simulink model "Anticipativo"  (R2018a)
settings: Solver=VariableStepAuto  StartTime=0.0  StopTime=1000  RelTol=1e-3
undefined symbols (not defined in the file or in its folder): Df1, Df2, Df4, Df5, Dgr, Dsmith, Nf1, Nf2, Nf4, Nf5, Ngr, Nsmith
settings Model: Creator=Dell  LastModifiedBy=Dell

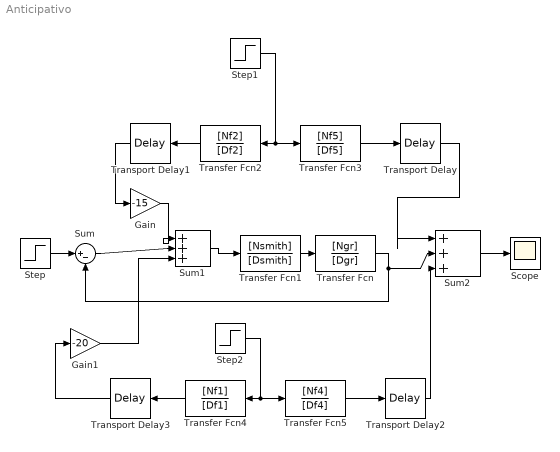
== system Anticipativo ==
  Gain : Gain  Gain=-15
  Gain1 : Gain  Gain=-20
  Scope : Scope
  Step : Step  Time=0  After=60  SampleTime=0
  Step1 : Step  Time=0  After=0.5  SampleTime=0
  Step2 : Step  Time=0  After=0.1  SampleTime=0
  Sum : Sum  Inputs=|+-
  Sum1 : Sum  Inputs=|+++
  Sum2 : Sum  Inputs=|+++
  Transfer Fcn : TransferFcn  Numerator=[Ngr]  Denominator=[Dgr]
  Transfer Fcn1 : TransferFcn  Numerator=[Nsmith]  Denominator=[Dsmith]
  Transfer Fcn2 : TransferFcn  Numerator=[Nf2]  Denominator=[Df2]
  Transfer Fcn3 : TransferFcn  Numerator=[Nf5]  Denominator=[Df5]
  Transfer Fcn4 : TransferFcn  Numerator=[Nf1]  Denominator=[Df1]
  Transfer Fcn5 : TransferFcn  Numerator=[Nf4]  Denominator=[Df4]
  Transport Delay : TransportDelay  DelayTime=300
  Transport Delay1 : TransportDelay  DelayTime=300
  Transport Delay2 : TransportDelay  DelayTime=600
  Transport Delay3 : TransportDelay  DelayTime=600
  wires:
  Transfer Fcn/1 -> Sum2/2, Sum/2
  Transfer Fcn1/1 -> Transfer Fcn/1
  Step/1 -> Sum/1
  Transfer Fcn3/1 -> Transport Delay/1
  Sum1/1 -> Transfer Fcn1/1
  Sum/1 -> Sum1/2
  Transfer Fcn2/1 -> Transport Delay1/1
  Step1/1 -> Transfer Fcn2/1, Transfer Fcn3/1
  Sum2/1 -> Scope/1
  Transport Delay/1 -> Sum2/1
  Step2/1 -> Transfer Fcn4/1, Transfer Fcn5/1
  Transfer Fcn5/1 -> Transport Delay2/1
  Transfer Fcn4/1 -> Transport Delay3/1
  Transport Delay2/1 -> Sum2/3
  Gain/1 -> Sum1/1
  Transport Delay1/1 -> Gain/1
  Transport Delay3/1 -> Gain1/1
  Gain1/1 -> Sum1/3
